simulink model "pitch_sim"  (R2021b)
settings: Solver=VariableStepAuto  StartTime=0.0  StopTime=20  RelTol=1e-3
values from neighbouring files (symbols this model uses):
  J_th = 1.1    [lab3_workspace.m]
  K_f = 0.0784    [lab3_workspace.m]
  K_th_d = ((J_th*(2*z_p*wn_p))/(K_f*l_a))    [lab3_workspace.m]
  K_th_i = 0.04*K_th_p    [lab3_workspace.m]
  K_th_p = ((J_th*wn_p^2)/(K_f*l_a))    [lab3_workspace.m]
  l_a = 0.63    [lab3_workspace.m]
settings Model: Creator=DSDLn  LastModifiedBy=DSDLn

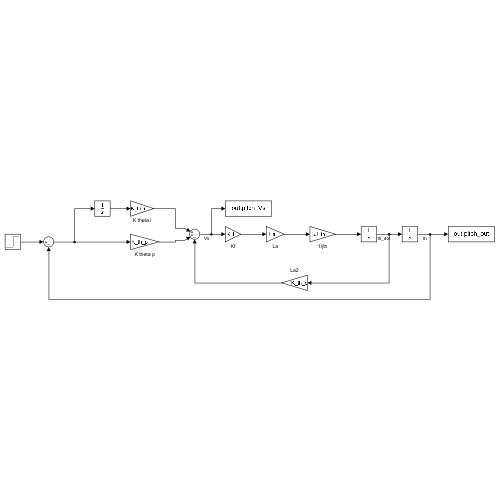
[thumbnail: Simulink's stored preview of the top-level diagram]
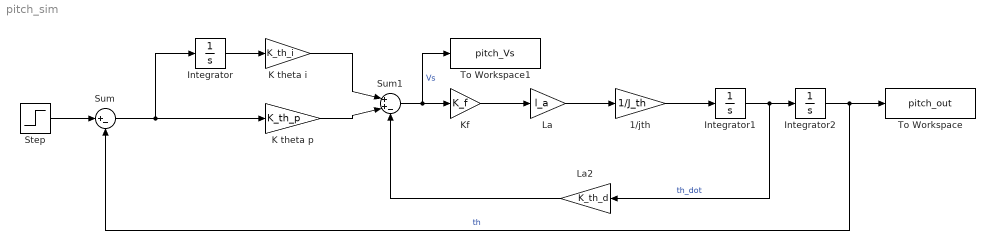
== system pitch_sim ==
  1/jth : Gain  Gain=1/J_th
  Integrator : Integrator
  Integrator1 : Integrator
  Integrator2 : Integrator
  K theta i : Gain  Gain=K_th_i
  K theta p : Gain  Gain=K_th_p
  Kf : Gain  Gain=K_f
  La : Gain  Gain=l_a
  La2 : Gain  Gain=K_th_d
  Step : Step  Time=0  After=deg2rad(20)  SampleTime=0.01
  Sum : Sum  Inputs=|+-
  Sum1 : Sum  Inputs=|++-
  To Workspace : ToWorkspace  VariableName=pitch_out  SampleTime=-1
  To Workspace1 : ToWorkspace  VariableName=pitch_Vs  SampleTime=-1
  wires:
  Integrator/1 -> K theta i/1
  Sum/1 -> K theta p/1, Integrator/1
  K theta p/1 -> Sum1/2
  K theta i/1 -> Sum1/1
  Sum1/1 -> To Workspace1/1, Kf/1  "Vs"
  Kf/1 -> La/1
  La/1 -> 1/jth/1
  1/jth/1 -> Integrator1/1
  Integrator1/1 -> Integrator2/1, La2/1  "th_dot"
  La2/1 -> Sum1/3
  Integrator2/1 -> To Workspace/1, Sum/2  "th"
  Step/1 -> Sum/1
